simulink model "withoutpfcbat"  (R2021a)
settings: Solver=VariableStepAuto  StartTime=0.0  StopTime=1  RelTol=1e-3
undefined symbols (not defined in the file): Ion, Lithium
libraries: spsDiodeLib x5, spsVoltageMeasurementLib x3, spsCurrentMeasurementLib x2, spsSeriesRLCBranchLib x2, spsACVoltageSourceLib x1, spsBatteryLib x1, spsMosfetLib x1, spspowerguiLib x1
settings Model: Creator=Jeyashree A  LastModifiedBy=Jeyashree A

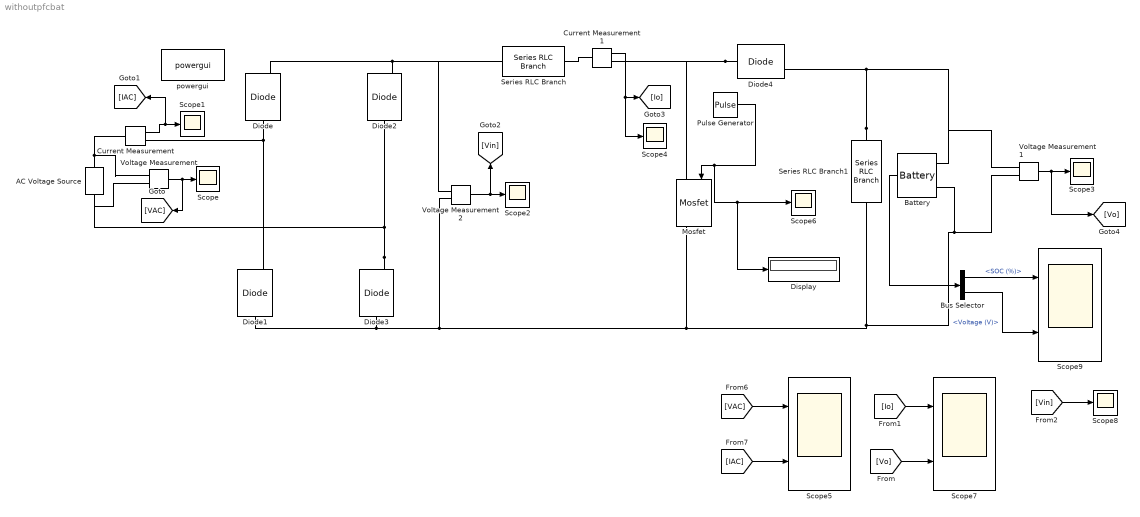
== system withoutpfcbat ==
  AC Voltage Source : spsACVoltageSourceLib/AC Voltage Source  Amplitude=325  Phase=0  Frequency=50  SampleTime=0  Measurements=None  BusType=swing  Pref=10e3  Qref=0  Qmin=-inf  Qmax=+inf
  Battery : spsBatteryLib/Battery  BatType=Lithium-Ion  ShowTempParam=off  ThermalPreset=no  ShowAgeParam=off  NomV=400  NomQ=5  SOC=20  Batt_Tr=30  PresetModel=on  MaxQ=5  MinV=300  FullV=465.5949  Dis_rate=2.1739  R=0.8  Normal_OP=4.5217  expZone="[432.1543     0.2456522]"  current=[6.5 13 32.5]  Units=Time  Tci=20  NomT=20  T2=-30  MaxQ2=4.8  FullV2=7.1  Normal_OP2=5.655  expZone2="[6.58           1]"  Rca=0.6  ti=2000  Dp=0  Neq0=0  Tsim=1e6  Ta1=25  Qeol=5.4*0.9  Reol=0.013333*1.2  Char_age=[2.3478, 3]  Dis_age=[2.3478, 10]  N1=1500  N2=10500  N3=1000  N4=1400  Ta2=45  N5=950
  Bus Selector : BusSelector  OutputSignals=SOC (%),Voltage (V)
  Current Measurement : spsCurrentMeasurementLib/Current Measurement  PhasorSimulation=off  OutputType=Complex  PSBequivalent=0
  Current Measurement1 : spsCurrentMeasurementLib/Current Measurement  PhasorSimulation=off  OutputType=Complex  PSBequivalent=0
  Diode{,1..4} (5 alike) : spsDiodeLib/Diode  Ron=0.001  Lon=0  Vf=0.8  IC=0  UseSnubber=0  Rs=500  Cs=250e-9  Measurements=on
  Display : Display
  Mosfet : spsMosfetLib/Mosfet  Ron=0.1  Lon=0  Rd=0.01  Vfd=0  IC=0  Rs=1e5  Cs=inf  Measurements=on
  Pulse Generator : DiscretePulseGenerator  PulseType=Time based  Period=(1/65000)  PulseWidth=50
  Scope{,1..4,6,8} (7 alike) : Scope
  Scope5 : Scope  NumInputPorts=2
  Scope7 : Scope  NumInputPorts=2
  Scope9 : Scope  NumInputPorts=2
  Series RLC Branch : spsSeriesRLCBranchLib/Series RLC Branch  LConnTagsString=__new0  RConnTagsString=__new0  BranchType=L  Resistance=1  Inductance=0.3e-3  SetiL0=off  InitialCurrent=0  Capacitance=1e-6  Setx0=off  InitialVoltage=0  Measurements=None
  Series RLC Branch1 : spsSeriesRLCBranchLib/Series RLC Branch  LConnTagsString=__new0  RConnTagsString=__new0  BranchType=C  Resistance=1  Inductance=1e-3  SetiL0=off  InitialCurrent=0  Capacitance=2000e-6  Setx0=off  InitialVoltage=0  Measurements=None
  Voltage Measurement : spsVoltageMeasurementLib/Voltage Measurement  PhasorSimulation=off  OutputType=Complex  PSBequivalent=0
  Voltage Measurement1 : spsVoltageMeasurementLib/Voltage Measurement  PhasorSimulation=off  OutputType=Complex  PSBequivalent=0
  Voltage Measurement2 : spsVoltageMeasurementLib/Voltage Measurement  PhasorSimulation=off  OutputType=Complex  PSBequivalent=0
  powergui : spspowerguiLib/powergui  Priority=1  SimulationMode=Discrete  SampleTime=1e-6  frequency=60  Iterations=50  frequencyindice=50  Pbase=100e6  ErrMax=1e-4  UnitsV=kV  UnitsW=MW  buscounter=0  FunctionMessages=off  echomessages=off  EnableUseOfTLC=off  CurrentSourceSwitches=off  DisableSnubberDevices=off  DisableRonSwitches=off  DisableVfSwitches=off  DisplayEquations=off  AutomaticDiscreteSolvers=off  SolverType=Tustin/Backward Euler (TBE)  Interpol=off  ExternalGateDelay=off  methode=off  Ts=100  x0status=blocks  SPID=on  SwTol=0  HookPort=off  NonlinearTolerance=1e-4  nMaxIteration=100  ContinueOnMaxIteration=off  RestoreLinks=warning  ResistiveCurrentMeasurement=off  Frange=[0:2:500]  Ylog=off  Xlog=on  ShowGrid=off  save=off  variable=ZData  structure=0  ZoomFFT=off  StartTime=0.0  cycles=1  DisplayStyle=1  fundamental=60  FreqAxis=off  MaxFrequency=1000  frequencyindicesteady=1  RmsSteady=1  display=off
  wires:
  Pulse Generator/1 -> Display/1, Scope6/1, Mosfet/1
  Current Measurement1/1 -> Scope4/1, [Io]
  Voltage Measurement1/1 -> [Vo], Scope3/1
  Voltage Measurement/1 -> [VAC], Scope/1
  [Io] -> Scope7/1
  [VAC] -> Scope5/1
  [IAC] -> Scope5/2
  Current Measurement/1 -> [IAC], Scope1/1
  Voltage Measurement2/1 -> [Vin], Scope2/1
  [Vin] -> Scope8/1
  [Vo] -> Scope7/2
  Battery/1 -> Bus Selector/1
  Bus Selector/1 -> Scope9/1  "<SOC (%)>"
  Bus Selector/2 -> Scope9/2  "<Voltage (V)>"
  connections:
  Diode/LConn1 -- Current Measurement/RConn1 -- Diode1/RConn1
  Diode2/RConn1 -- Voltage Measurement2/LConn1 -- Series RLC Branch/LConn1 -- Diode/RConn1
  Voltage Measurement1/LConn2 -- Battery/LConn2 -- Series RLC Branch1/RConn1 -- Mosfet/RConn1 -- Voltage Measurement2/LConn2 -- Diode1/LConn1 -- Diode3/LConn1
  Series RLC Branch1/LConn1 -- Battery/LConn1 -- Voltage Measurement1/LConn1 -- Diode4/RConn1
  Diode4/LConn1 -- Mosfet/LConn1 -- Current Measurement1/RConn1
  AC Voltage Source/RConn1 -- Current Measurement/LConn1 -- Voltage Measurement/LConn1
  Diode3/RConn1 -- AC Voltage Source/LConn1 -- Voltage Measurement/LConn2 -- Diode2/LConn1
  Current Measurement1/LConn1 -- Series RLC Branch/RConn1
